simulink model "Linearisierung3_RoboMotor_Sim"  (R2017a)
settings: Solver=VariableStepAuto  StartTime=0.0  StopTime=10.0  RelTol=1e-3
values from neighbouring files (symbols this model uses):
  K = 300    [Linearisierung3_Robo.m]
  T = 0.1    [Linearisierung3_Robo.m]
settings Model: Creator=Jonas  LastModifiedBy=jonas

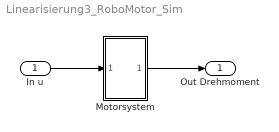
== system Linearisierung3_RoboMotor_Sim ==
  "In u " : Inport
  Motorsystem : Subsystem
  Out Drehmoment : Outport
  wires:
  "In u "/1 -> Motorsystem/1("In u ")
  Motorsystem/1(Out Drehmoment) -> Out Drehmoment/1

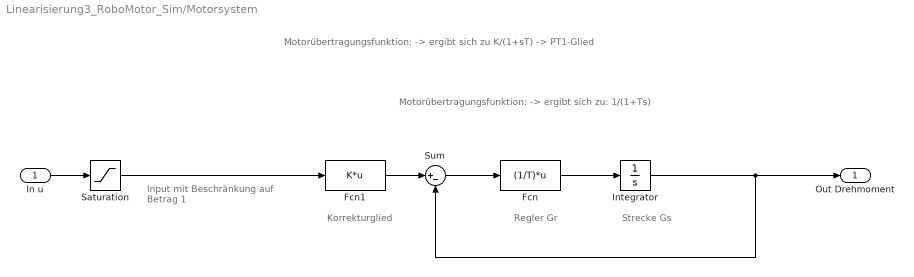
== system Linearisierung3_RoboMotor_Sim/Motorsystem ==
  note: Motorübertragungsfunktion:
      |  -> ergibt sich zu K/(1+sT)
      |  -> PT1-Glied
  note: Motorübertragungsfunktion:
      |  -> ergibt sich zu: 1/(1+Ts)
  note: Korrekturglied
  note: Input
      | mit Beschränkung
      | auf Betrag 1
  note: Regler Gr
  note: Strecke Gs
  "In u " : Inport
  Fcn : Fcn  Expr=(1/T)*u
  Fcn1 : Fcn  Expr=K*u
  Integrator : Integrator
  Saturation : Saturate  UpperLimit=1  LowerLimit=-1
  Sum : Sum  Inputs=|+-
  Out Drehmoment : Outport
  wires:
  Fcn1/1 -> Sum/1
  Fcn/1 -> Integrator/1
  Integrator/1 -> Out Drehmoment/1, Sum/2
  "In u "/1 -> Saturation/1
  Saturation/1 -> Fcn1/1
  Sum/1 -> Fcn/1
